simulink library "VEH_CAN"  (R2017a)
settings: Solver=VariableStepAuto  StartTime=0.0  StopTime=10.0  RelTol=1e-3
settings Model: Creator=Di Russo  LastModifiedBy=Vraj M

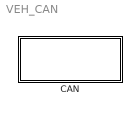
== system VEH_CAN ==
  CAN : Subsystem

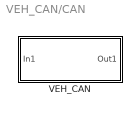
== system VEH_CAN/CAN ==
  VEH_CAN : Subsystem

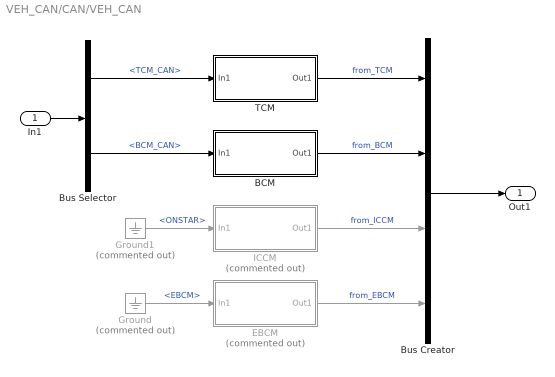
== system VEH_CAN/CAN/VEH_CAN ==
  In1 : Inport
  BCM : Subsystem
  Bus Creator : BusCreator  Inputs=4
  Bus Selector : BusSelector  OutputSignals=TCM_CAN,BCM_CAN
  EBCM : Subsystem  Commented=on
  Ground : Ground  Commented=on
  Ground1 : Ground  Commented=on
  ICCM : Subsystem  Commented=on
  TCM : Subsystem
  Out1 : Outport
  wires:
  In1/1 -> Bus Selector/1
  TCM/1(Out1) -> Bus Creator/1  "from_TCM"
  BCM/1(Out1) -> Bus Creator/2  "from_BCM"
  ICCM/1(Out1) -> Bus Creator/3  "from_ICCM"
  EBCM/1(Out1) -> Bus Creator/4  "from_EBCM"
  Bus Creator/1 -> Out1/1
  Bus Selector/1 -> TCM/1(In1)  "<TCM_CAN>"
  Bus Selector/2 -> BCM/1(In1)  "<BCM_CAN>"
  Ground1/1 -> ICCM/1(In1)  "<ONSTAR>"
  Ground/1 -> EBCM/1(In1)  "<EBCM>"

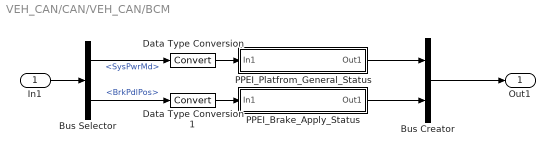
== system VEH_CAN/CAN/VEH_CAN/BCM ==
  In1 : Inport
  Bus Creator : BusCreator  Inputs=2
  Bus Selector : BusSelector  OutputSignals=SysPwrMd,BrkPdlPos
  Data Type Conversion : DataTypeConversion
  Data Type Conversion1 : DataTypeConversion
  PPEI_Brake_Apply_Status : Subsystem
  PPEI_Platfrom_General_Status : Subsystem
  Out1 : Outport
  wires:
  In1/1 -> Bus Selector/1
  Bus Selector/1 -> Data Type Conversion/1  "<SysPwrMd>"
  Bus Selector/2 -> Data Type Conversion1/1  "<BrkPdlPos>"
  PPEI_Platfrom_General_Status/1(Out1) -> Bus Creator/1
  PPEI_Brake_Apply_Status/1(Out1) -> Bus Creator/2
  Bus Creator/1 -> Out1/1
  Data Type Conversion/1 -> PPEI_Platfrom_General_Status/1(In1)
  Data Type Conversion1/1 -> PPEI_Brake_Apply_Status/1(In1)

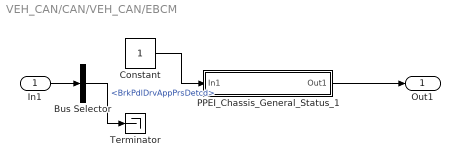
== system VEH_CAN/CAN/VEH_CAN/EBCM ==
  In1 : Inport
  Bus Selector : BusSelector  OutputSignals=PPEI_Chassis_General_Status_1.BrkPdlDrvAppPrsDetcd
  Constant : Constant  OutDataTypeStr=boolean
  PPEI_Chassis_General_Status_1 : Subsystem
  Terminator : Terminator
  Out1 : Outport
  wires:
  Bus Selector/1 -> Terminator/1  "<BrkPdlDrvAppPrsDetcd>"
  PPEI_Chassis_General_Status_1/1(Out1) -> Out1/1
  In1/1 -> Bus Selector/1
  Constant/1 -> PPEI_Chassis_General_Status_1/1(In1)

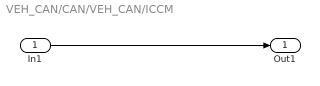
== system VEH_CAN/CAN/VEH_CAN/ICCM ==
  In1 : Inport
  Out1 : Outport
  wires:
  In1/1 -> Out1/1

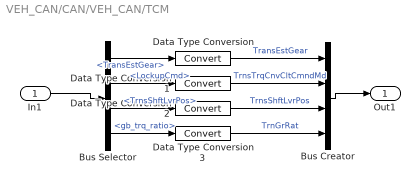
== system VEH_CAN/CAN/VEH_CAN/TCM ==
  In1 : Inport
  Bus Creator : BusCreator  Inputs=4
  Bus Selector : BusSelector  OutputSignals=TCM_to _Actuator.TransEstGear,TCM_to _Actuator.LockupCmd,TCM_to _Actuator.TrnsShftLvrPos,Sensors_to_TCM.gb_trq_ratio
  Data Type Conversion{,1..3} (4 alike) : DataTypeConversion
  Out1 : Outport
  wires:
  Bus Selector/4 -> Data Type Conversion3/1  "<gb_trq_ratio>"
  Bus Selector/3 -> Data Type Conversion2/1  "<TrnsShftLvrPos>"
  Bus Selector/2 -> Data Type Conversion1/1  "<LockupCmd>"
  Bus Selector/1 -> Data Type Conversion/1  "<TransEstGear>"
  Data Type Conversion3/1 -> Bus Creator/4  "TrnGrRat"
  Data Type Conversion2/1 -> Bus Creator/3  "TrnsShftLvrPos"
  Data Type Conversion1/1 -> Bus Creator/2  "TrnsTrqCnvCltCmndMd"
  In1/1 -> Bus Selector/1
  Bus Creator/1 -> Out1/1
  Data Type Conversion/1 -> Bus Creator/1  "TransEstGear"

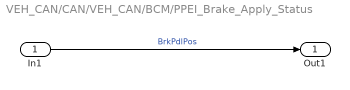
== system VEH_CAN/CAN/VEH_CAN/BCM/PPEI_Brake_Apply_Status ==
  In1 : Inport
  Out1 : Outport
  wires:
  In1/1 -> Out1/1  "BrkPdlPos"

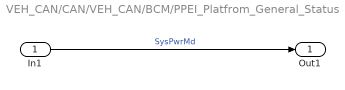
== system VEH_CAN/CAN/VEH_CAN/BCM/PPEI_Platfrom_General_Status ==
  In1 : Inport
  Out1 : Outport
  wires:
  In1/1 -> Out1/1  "SysPwrMd"

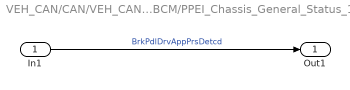
== system VEH_CAN/CAN/VEH_CAN/EBCM/PPEI_Chassis_General_Status_1 ==
  In1 : Inport
  Out1 : Outport
  wires:
  In1/1 -> Out1/1  "BrkPdlDrvAppPrsDetcd"
